simulink library "contractLibs"  (R2019b)
settings: Solver=VariableStepAuto  StartTime=0.0  StopTime=10.0  RelTol=1e-3
undefined symbols (not defined in the file or in its folder): ContractAssumeBlock, ContractBlock, ContractGuaranteeBlock, ContractModeBlock, ContractValidatorBlock
libraries: cocosimLibs x5
settings Model: Creator=hbourbou  LastModifiedBy=hbourbou
settings DataIOCC: ReturnWorkspaceOutputs=off
settings DebuggingCC: ArithmeticOperatorsInVariantConditions=warning
settings SFSimCC: SimUseLocalCustomCode=off  CustomCodeUndefinedFunction=UseInterfaceOnly
settings RTWCC: RTWUseLocalCustomCode=off

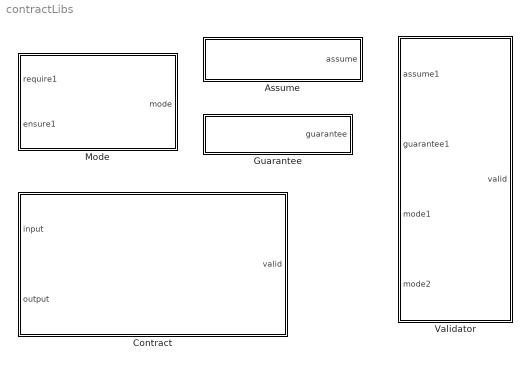
== system contractLibs ==
  Assume : Subsystem  mask(ContractAssumeBlock){ContractBlockType=ContractAssumeBlock}
      mask init:
      | set_param(gcb, 'LinkStatus', 'none');
      mask DialogControl DescTextVar Prompt: Assume block
      mask Display: text(0.5, 0.5, '{\bf\fontsize{20}Assume}', 'hor', 'center', 'texmode','on');
  Contract : Subsystem  mask(ContractBlock){ContractBlockType=ContractBlock, ShowInLibBrowser=on}
      mask init:
      | set_param(gcb, 'LinkStatus', 'none');
      settings: CopyFcn=set_param(gcb, 'LinkStatus', 'none');
      mask DialogControl DescTextVar Prompt: Contract block
      mask Display: text(0.5, 0.5, '{\bf\fontsize{20}Contract}', 'hor', 'center', 'texmode','on');
  Guarantee : Subsystem  mask(ContractGuaranteeBlock){ContractBlockType=ContractGuaranteeBlock}
      mask init:
      | set_param(gcb, 'LinkStatus', 'none');
      mask DialogControl DescTextVar Prompt: Guarantee block
      mask Display: text(0.5, 0.5, '{\bf\fontsize{20}Guarantee}', 'hor', 'center', 'texmode','on');
  Mode : Subsystem  mask(ContractModeBlock){requirePorts=1, ensurePorts=1, ContractBlockType=ContractModeBlock}
      mask prompts: requirePorts "Require ports     :"; ensurePorts "Ensure ports     :"
      mask init:
      | set_param(gcb, 'LinkStatus', 'none');
      | coco_blockCallbacks.CoCoSimContract.modeCallback(gcb);
      mask Display: disp('Mode: \n(require1 && require2 ..)\n =>\n (ensure1 && ensure2 ..)')
  Validator : Subsystem  mask(ContractValidatorBlock){assumePorts=1, guaranteePorts=1, modePorts=2, ContractBlockType=ContractValidatorBlock}
      mask prompts: assumePorts "Assume ports     :"; guaranteePorts "Guarantee ports :"; modePorts "Mode ports        :"
      mask help: The validator block implements the following logic: <br> <br> <b>Sofar</b>(assume<sub>1</sub> <b>&#8743;</b> assume<sub>2</sub> <b>&#8743;</b> ... assume<sub>k</sub>) <b>&rarr;</b> <b>Sofar</b>(guarantee<sub>1</sub> <b>&#8743;</b> guarantee<sub>2</sub> <b>&#8743;</b> ... guarantee<sub>m</sub> <b>&#8743;</b> mode<sub>1</sub> <b>&#8743;</b> mode<sub>2</sub> <b>&#8743;</b> ... <b>&#8743;</b> mode<sub>n</sub> )<br> where mode<sub>i</sub> = require<sub>i</sub> <b>&rarr;</b> ensure<sub>i</sub>
      mask init:
      | set_param(gcb,'LinkStatus','none');
      | coco_blockCallbacks.CoCoSimContract.validatorCallback(gcb);
      mask Display: disp(' ')

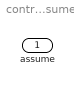
== system contractLibs/Assume ==
  assume : Outport  OutDataTypeStr=boolean  VectorParamsAs1DForOutWhenUnconnected=off

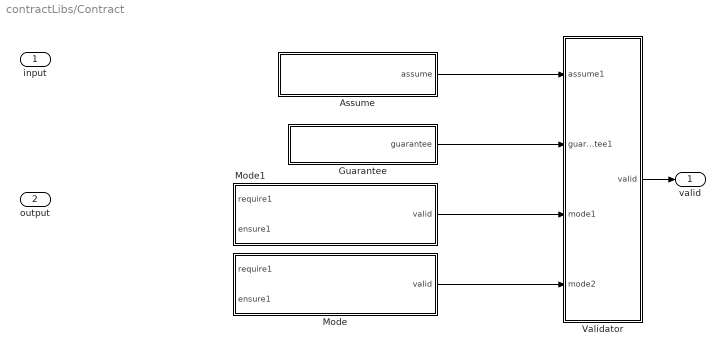
== system contractLibs/Contract ==
  input : Inport
  output : Inport  Port=2
  Assume : Subsystem  mask(ContractAssumeBlock){ContractBlockType=ContractAssumeBlock}
      mask init:
      | set_param(gcb, 'LinkStatus', 'none');
      mask DialogControl DescTextVar Prompt: Assume block
      mask Display: text(0.5, 0.5, '{\bf\fontsize{20}Assume}', 'hor', 'center', 'texmode','on');
  Guarantee : Subsystem  mask(ContractGuaranteeBlock){ContractBlockType=ContractGuaranteeBlock}
      mask init:
      | set_param(gcb, 'LinkStatus', 'none');
      mask DialogControl DescTextVar Prompt: Guarantee block
      mask Display: text(0.5, 0.5, '{\bf\fontsize{20}Guarantee}', 'hor', 'center', 'texmode','on');
  Mode : Subsystem  mask(ContractModeBlock){requirePorts=1, ensurePorts=1, ContractBlockType=ContractModeBlock}
      mask prompts: requirePorts "Require ports     :"; ensurePorts "Ensure ports     :"
      mask init:
      | set_param(gcb, 'LinkStatus', 'none');
      | coco_blockCallbacks.CoCoSimContract.modeCallback(gcb);
      mask Display: disp('Mode: \n(require1 && require2 ..)\n =>\n (ensure1 && ensure2 ..)')
  Mode1 : Subsystem  mask(ContractModeBlock){requirePorts=1, ensurePorts=1, ContractBlockType=ContractModeBlock}
      mask prompts: requirePorts "Require ports     :"; ensurePorts "Ensure ports     :"
      mask init:
      | set_param(gcb, 'LinkStatus', 'none');
      | coco_blockCallbacks.CoCoSimContract.modeCallback(gcb);
      mask Display: disp('Mode: \n(require1 && require2 ..)\n =>\n (ensure1 && ensure2 ..)')
  Validator : Subsystem  mask(ContractValidatorBlock){assumePorts=1, guaranteePorts=1, modePorts=2, ContractBlockType=ContractValidatorBlock}
      mask prompts: assumePorts "Assume ports     :"; guaranteePorts "Guarantee ports :"; modePorts "Mode ports        :"
      mask help: The validator block implements the following logic: <br> <br> <b>Sofar</b>(assume<sub>1</sub> <b>&#8743;</b> assume<sub>2</sub> <b>&#8743;</b> ... assume<sub>k</sub>) <b>&rarr;</b> <b>Sofar</b>(guarantee<sub>1</sub> <b>&#8743;</b> guarantee<sub>2</sub> <b>&#8743;</b> ... guarantee<sub>m</sub> <b>&#8743;</b> mode<sub>1</sub> <b>&#8743;</b> mode<sub>2</sub> <b>&#8743;</b> ... <b>&#8743;</b> mode<sub>n</sub> )<br> where mode<sub>i</sub> = require<sub>i</sub> <b>&rarr;</b> ensure<sub>i</sub>
      mask init:
      | set_param(gcb,'LinkStatus','none');
      | coco_blockCallbacks.CoCoSimContract.validatorCallback(gcb);
      mask Display: disp(' ')
  valid : Outport  VectorParamsAs1DForOutWhenUnconnected=off
  wires:
  Validator/1(valid) -> valid/1
  Mode/1(valid) -> Validator/4(mode2)
  Mode1/1(valid) -> Validator/3(mode1)
  Assume/1(assume) -> Validator/1(assume1)
  Guarantee/1(guarantee) -> Validator/2(guarantee1)

== system contractLibs/Guarantee ==
  guarantee : Outport  OutDataTypeStr=boolean  VectorParamsAs1DForOutWhenUnconnected=off

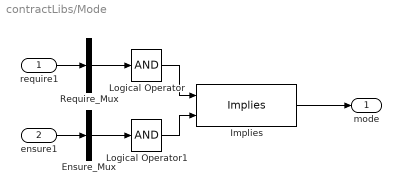
== system contractLibs/Mode ==
  require1 : Inport  OutDataTypeStr=boolean  PortDimensions=1
  ensure1 : Inport  Port=2  OutDataTypeStr=boolean  PortDimensions=1
  Ensure_Mux : Mux  Inputs=1
  Implies : cocosimLibs/Implies  SystemSampleTime=-1
      settings: SourceProductName=CoCoSim Specification Library
  Logical Operator : Logic  Inputs=1  AllPortsSameDT=off  OutDataTypeStr=boolean
  Logical Operator1 : Logic  Inputs=1  AllPortsSameDT=off  OutDataTypeStr=boolean
  Require_Mux : Mux  Inputs=1
  mode : Outport  VectorParamsAs1DForOutWhenUnconnected=off
  wires:
  ensure1/1 -> Ensure_Mux/1
  require1/1 -> Require_Mux/1
  Ensure_Mux/1 -> Logical Operator1/1
  Logical Operator1/1 -> Implies/2
  Logical Operator/1 -> Implies/1
  Require_Mux/1 -> Logical Operator/1
  Implies/1 -> mode/1

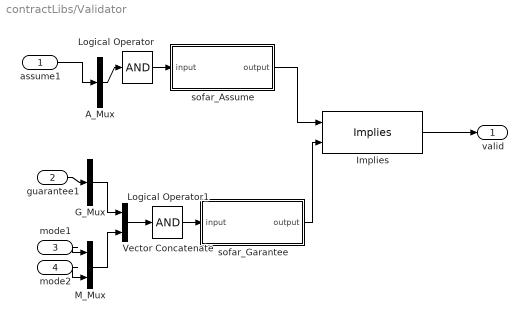
== system contractLibs/Validator ==
  assume1 : Inport  OutDataTypeStr=boolean  PortDimensions=1
  guarantee1 : Inport  Port=2  OutDataTypeStr=boolean  PortDimensions=1
  mode1 : Inport  Port=3  OutDataTypeStr=boolean  PortDimensions=1
  mode2 : Inport  Port=4  OutDataTypeStr=boolean  PortDimensions=1
  A_Mux : Mux  Inputs=1
  G_Mux : Mux  Inputs=1
  Implies : cocosimLibs/Implies  SystemSampleTime=-1
      settings: SourceProductName=CoCoSim Specification Library
  Logical Operator : Logic  Inputs=1  AllPortsSameDT=off  OutDataTypeStr=boolean
  Logical Operator1 : Logic  Inputs=1  AllPortsSameDT=off  OutDataTypeStr=boolean
  M_Mux : Mux  Inputs=2
  Vector Concatenate : Concatenate
  sofar_Assume : Subsystem
  sofar_Garantee : Subsystem
  valid : Outport  VectorParamsAs1DForOutWhenUnconnected=off
  wires:
  mode2/1 -> M_Mux/2
  mode1/1 -> M_Mux/1
  M_Mux/1 -> Vector Concatenate/2
  Vector Concatenate/1 -> Logical Operator1/1
  assume1/1 -> A_Mux/1
  guarantee1/1 -> G_Mux/1
  G_Mux/1 -> Vector Concatenate/1
  Logical Operator1/1 -> sofar_Garantee/1(input)
  Logical Operator/1 -> sofar_Assume/1(input)
  A_Mux/1 -> Logical Operator/1
  Implies/1 -> valid/1
  sofar_Garantee/1(output) -> Implies/2
  sofar_Assume/1(output) -> Implies/1

== system contractLibs/Contract/Assume ==
  assume : Outport  OutDataTypeStr=boolean  VectorParamsAs1DForOutWhenUnconnected=off

== system contractLibs/Contract/Guarantee ==
  guarantee : Outport  OutDataTypeStr=boolean  VectorParamsAs1DForOutWhenUnconnected=off

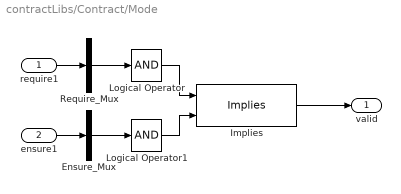
== system contractLibs/Contract/Mode ==
  require1 : Inport  OutDataTypeStr=boolean  PortDimensions=1
  ensure1 : Inport  Port=2  OutDataTypeStr=boolean  PortDimensions=1
  Ensure_Mux : Mux  Inputs=1
  Implies : cocosimLibs/Implies  SystemSampleTime=-1
      settings: SourceProductName=CoCoSim Specification Library
  Logical Operator : Logic  Inputs=1  AllPortsSameDT=off  OutDataTypeStr=boolean
  Logical Operator1 : Logic  Inputs=1  AllPortsSameDT=off  OutDataTypeStr=boolean
  Require_Mux : Mux  Inputs=1
  valid : Outport  VectorParamsAs1DForOutWhenUnconnected=off
  wires:
  ensure1/1 -> Ensure_Mux/1
  require1/1 -> Require_Mux/1
  Ensure_Mux/1 -> Logical Operator1/1
  Logical Operator1/1 -> Implies/2
  Logical Operator/1 -> Implies/1
  Require_Mux/1 -> Logical Operator/1
  Implies/1 -> valid/1

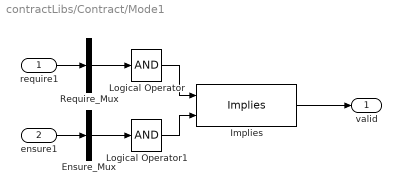
== system contractLibs/Contract/Mode1 ==
  require1 : Inport  OutDataTypeStr=boolean  PortDimensions=1
  ensure1 : Inport  Port=2  OutDataTypeStr=boolean  PortDimensions=1
  Ensure_Mux : Mux  Inputs=1
  Implies : cocosimLibs/Implies  SystemSampleTime=-1
      settings: SourceProductName=CoCoSim Specification Library
  Logical Operator : Logic  Inputs=1  AllPortsSameDT=off  OutDataTypeStr=boolean
  Logical Operator1 : Logic  Inputs=1  AllPortsSameDT=off  OutDataTypeStr=boolean
  Require_Mux : Mux  Inputs=1
  valid : Outport  VectorParamsAs1DForOutWhenUnconnected=off
  wires:
  ensure1/1 -> Ensure_Mux/1
  require1/1 -> Require_Mux/1
  Ensure_Mux/1 -> Logical Operator1/1
  Logical Operator1/1 -> Implies/2
  Logical Operator/1 -> Implies/1
  Require_Mux/1 -> Logical Operator/1
  Implies/1 -> valid/1

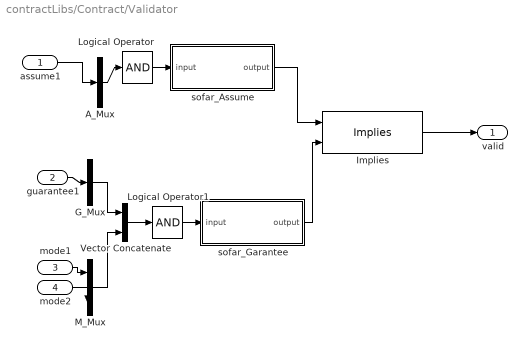
== system contractLibs/Contract/Validator ==
  assume1 : Inport  OutDataTypeStr=boolean  PortDimensions=1
  guarantee1 : Inport  Port=2  OutDataTypeStr=boolean  PortDimensions=1
  mode1 : Inport  Port=3  OutDataTypeStr=boolean  PortDimensions=1
  mode2 : Inport  Port=4  OutDataTypeStr=boolean  PortDimensions=1
  A_Mux : Mux  Inputs=1
  G_Mux : Mux  Inputs=1
  Implies : cocosimLibs/Implies  SystemSampleTime=-1
      settings: SourceProductName=CoCoSim Specification Library
  Logical Operator : Logic  Inputs=1  AllPortsSameDT=off  OutDataTypeStr=boolean
  Logical Operator1 : Logic  Inputs=1  AllPortsSameDT=off  OutDataTypeStr=boolean
  M_Mux : Mux  Inputs=2
  Vector Concatenate : Concatenate
  sofar_Assume : Subsystem
  sofar_Garantee : Subsystem
  valid : Outport  VectorParamsAs1DForOutWhenUnconnected=off
  wires:
  sofar_Assume/1(output) -> Implies/1
  sofar_Garantee/1(output) -> Implies/2
  Implies/1 -> valid/1
  A_Mux/1 -> Logical Operator/1
  Logical Operator/1 -> sofar_Assume/1(input)
  Logical Operator1/1 -> sofar_Garantee/1(input)
  G_Mux/1 -> Vector Concatenate/1
  guarantee1/1 -> G_Mux/1
  assume1/1 -> A_Mux/1
  Vector Concatenate/1 -> Logical Operator1/1
  M_Mux/1 -> Vector Concatenate/2
  mode1/1 -> M_Mux/1
  mode2/1 -> M_Mux/2

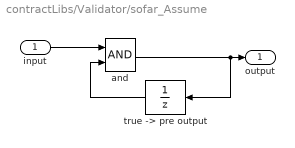
== system contractLibs/Validator/sofar_Assume ==
  input : Inport  OutDataTypeStr=boolean
  and : Logic  AllPortsSameDT=off  OutDataTypeStr=boolean
  "true -> pre output" : UnitDelay  InitialCondition=true  SampleTime=-1  HasFrameUpgradeWarning=on
  output : Outport  OutDataTypeStr=boolean  VectorParamsAs1DForOutWhenUnconnected=off
  wires:
  and/1 -> output/1, "true -> pre output"/1
  "true -> pre output"/1 -> and/2
  input/1 -> and/1

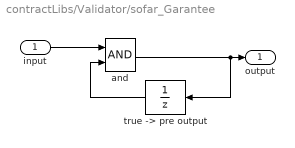
== system contractLibs/Validator/sofar_Garantee ==
  input : Inport  OutDataTypeStr=boolean
  and : Logic  AllPortsSameDT=off  OutDataTypeStr=boolean
  "true -> pre output" : UnitDelay  InitialCondition=true  SampleTime=-1  HasFrameUpgradeWarning=on
  output : Outport  OutDataTypeStr=boolean  VectorParamsAs1DForOutWhenUnconnected=off
  wires:
  and/1 -> output/1, "true -> pre output"/1
  "true -> pre output"/1 -> and/2
  input/1 -> and/1

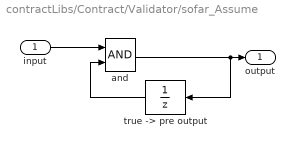
== system contractLibs/Contract/Validator/sofar_Assume ==
  input : Inport  OutDataTypeStr=boolean
  and : Logic  AllPortsSameDT=off  OutDataTypeStr=boolean
  "true -> pre output" : UnitDelay  InitialCondition=true  SampleTime=-1  HasFrameUpgradeWarning=on
  output : Outport  OutDataTypeStr=boolean  VectorParamsAs1DForOutWhenUnconnected=off
  wires:
  input/1 -> and/1
  "true -> pre output"/1 -> and/2
  and/1 -> "true -> pre output"/1, output/1

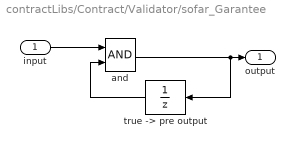
== system contractLibs/Contract/Validator/sofar_Garantee ==
  input : Inport  OutDataTypeStr=boolean
  and : Logic  AllPortsSameDT=off  OutDataTypeStr=boolean
  "true -> pre output" : UnitDelay  InitialCondition=true  SampleTime=-1  HasFrameUpgradeWarning=on
  output : Outport  OutDataTypeStr=boolean  VectorParamsAs1DForOutWhenUnconnected=off
  wires:
  input/1 -> and/1
  "true -> pre output"/1 -> and/2
  and/1 -> "true -> pre output"/1, output/1
